simulink model "Env"  (R2020a)
settings: Solver=VariableStepAuto  StartTime=0.0  StopTime=10.0  RelTol=1e-3
settings Model: Creator=Administrator  LastModifiedBy=Administrator

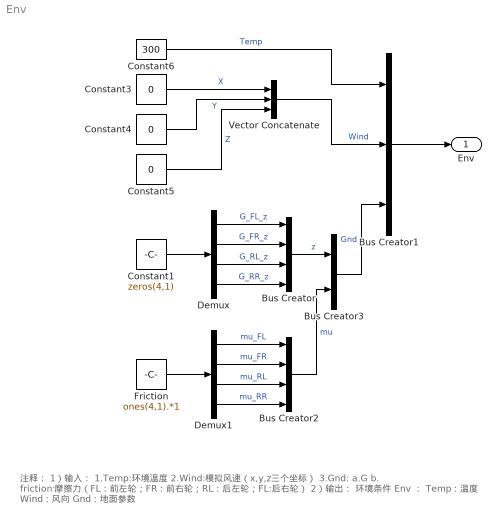
== system Env ==
  note: 注释：
      | 1）输入：
      | 1.Temp:环境温度
      | 2.Wind:模拟风速（x,y,z三个坐标）
      | 3.Gnd: a.G
      | b. friction:摩擦力（FL：前左轮；FR：前右轮；RL：后左轮；FL:后右轮）
      |
      | 2）输出：
      | 环境条件 Env ：
      | Temp：温度
      | Wind：风向
      | Gnd：地面参数
  Bus Creator : BusCreator  Inputs=4
  Bus Creator1 : BusCreator  Inputs=3
  Bus Creator2 : BusCreator  Inputs=4
  Bus Creator3 : BusCreator  Inputs=2
  Constant1 : Constant  Value=zeros(4,1)
  Constant3 : Constant  Value=0
  Constant4 : Constant  Value=0
  Constant5 : Constant  Value=0
  Constant6 : Constant  Value=300
  Demux : Demux
  Demux1 : Demux
  Friction : Constant  Value=ones(4,1).*1
  Vector Concatenate : Concatenate  NumInputs=3
  Env : Outport  VectorParamsAs1DForOutWhenUnconnected=off
  wires:
  Bus Creator1/1 -> Env/1
  Constant6/1 -> Bus Creator1/1  "Temp"
  Constant5/1 -> Vector Concatenate/3  "Z"
  Demux1/3 -> Bus Creator2/3  "mu_RL"
  Friction/1 -> Demux1/1
  Vector Concatenate/1 -> Bus Creator1/2  "Wind"
  Demux1/2 -> Bus Creator2/2  "mu_FR"
  Demux1/1 -> Bus Creator2/1  "mu_FL"
  Demux1/4 -> Bus Creator2/4  "mu_RR"
  Constant4/1 -> Vector Concatenate/2  "Y"
  Bus Creator2/1 -> Bus Creator3/2  "mu"
  Constant3/1 -> Vector Concatenate/1  "X"
  Demux/3 -> Bus Creator/3  "G_RL_z"
  Demux/4 -> Bus Creator/4  "G_RR_z"
  Demux/2 -> Bus Creator/2  "G_FR_z"
  Bus Creator/1 -> Bus Creator3/1  "z"
  Constant1/1 -> Demux/1
  Demux/1 -> Bus Creator/1  "G_FL_z"
  Bus Creator3/1 -> Bus Creator1/3  "Gnd"
